simulink model "DRPLDM"  (R2019a)
settings: Solver=FixedStepAuto  StartTime=0.0  StopTime=TimeVector(end)  FixedStep=Tsim  RelTol=1e-3  EnableMultiTasking=on
values from neighbouring files (symbols this model uses):
  Ad = 0.9048    [RunModel.m]
  B1DELTT = [1 100 130]    [RunModel.m]
  B1ERPM = [0 20000 23000]    [RunModel.m]
  B1NOOILT = [300 450 573]    [RunModel.m]
  B2DELTT = [1 40 120]    [RunModel.m]
  B2ERPM = [0 20000 23000]    [RunModel.m]
  B2NOOILT = [300 400 530]    [RunModel.m]
  B3DELTT = [1 50 110]    [RunModel.m]
  B3ERPM = [0 20000 23000]    [RunModel.m]
  B3NOOILT = [300 410 540]    [RunModel.m]
  Bd = 0.1903    [RunModel.m]
  BoosterVec = [hex2dec('55'), hex2dec('AA') hex2dec('FF')]    [RunModel.m]
  Cd = -0.5    [RunModel.m]
  Dd = 0    [RunModel.m]
  DigKeys = bin2dec('0101011')    [RunModel.m]
  EngUnits = 1    [RunModel.m]
  ExComTime = ExComTime + DeltaTimeEnd    [RunModel.m]
  ExComVec = [hex2dec('AA'), hex2dec('00'), hex2dec('CC')]    [RunModel.m]
  ExtFPModel = 0    [RunModel.m]
  FlightStart = 0    [RunModel.m]
  HILMode = 1    [RunModel.m]
  LeverMode = 1    [RunModel.m]
  Mode = 0    [RunModel.m]
  Mwm = 0.35    [RunModel.m]
  OPRPMMax = 4500    [RunModel.m]
  SensFaultStartTime = SensFaultStartTime + DeltaTimeEnd    [RunModel.m]
  SensFaultStopTime = SensFaultStopTime + DeltaTimeEnd    [RunModel.m]
  SysFaultStartTime = SysFaultStartTime + DeltaTimeEnd    [RunModel.m]
  SysFaultStopTime = SysFaultStopTime + DeltaTimeEnd    [RunModel.m]
  TBear1Init = 0    [RunModel.m]
  TBear2Init = 0    [RunModel.m]
  TBear3Init = 0    [RunModel.m]
  Tsim = 0.001 * TICK    [RunModel.m]
  WhichCont = 2    [RunModel.m]
  WhichEngine = 1    [RunModel.m]
undefined symbols (not defined in the file or in its folder): BiasSens, BoosterLStatusTime, BoosterRStatusTime
libraries: Lib_Solve_ModelSource_TMATS x5, simulink x5
(part 1 of 2)
settings Model: Creator=antoniohadadeneto  LastModifiedBy=anton
settings DataIOCC: ReturnWorkspaceOutputs=off
settings OptimizationCC: LifeSpan=inf
settings DebuggingCC: AllowSymbolicDim=off  SFUnexpectedBacktrackingDiag=warning  SFNoUnconditionalDefaultTransitionDiag=warning  SFExecutionAtInitializationDiag=none  ArithmeticOperatorsInVariantConditions=warning
settings ModelReferenceCC: PropagateSignalLabelsOutOfModel=off
settings SFSimCC: SimUseLocalCustomCode=off
settings RTWCC: RTWUseLocalCustomCode=off
settings CodeAppCC: StateflowObjectComments=on
settings GRTTargetCC: TargetLangStandard=C89/C90 (ANSI)
settings ConfigComp: CovMetricSettings=dw  CovHtmlReporting=on  CovSaveCumulativeToWorkspaceVar=on  CovSaveSingleToWorkspaceVar=on  CovExternalEMLEnable=off

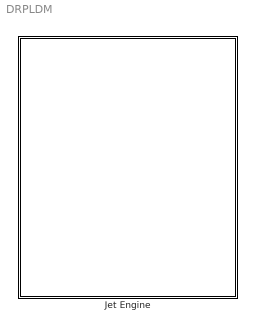
== system DRPLDM ==
  Jet Engine : Subsystem

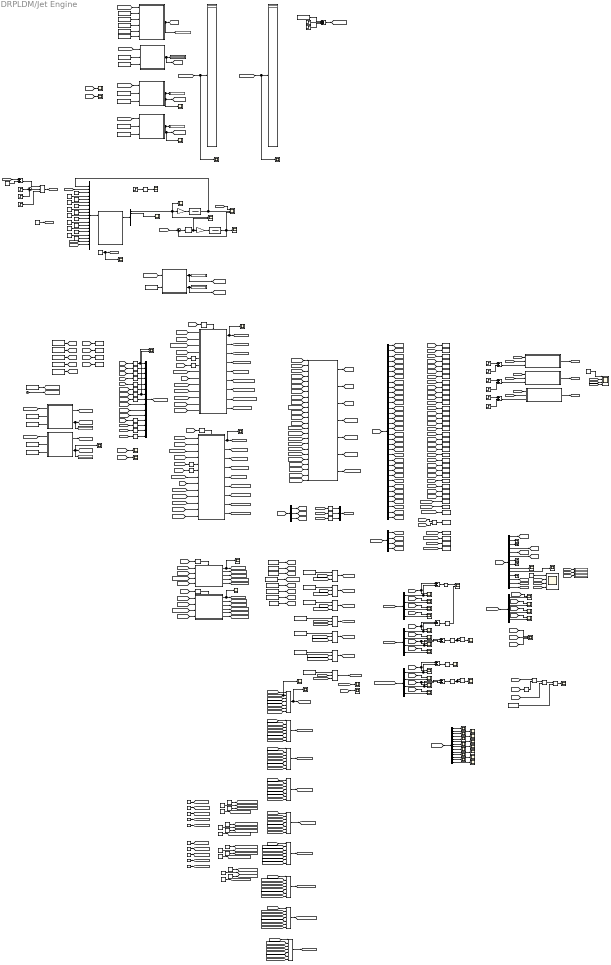
== system DRPLDM/Jet Engine ==
  note: SysFaultTime positions for Emergency and Shut Off respectively
  note: Vector Inputs
  note: Single Spoo Engine
      | Piecewise
      | Linear Model
  note: Bearings Models
  note: Output Selectors
  note: FADEC
  note: To Workspace
  Abnormal DeltaT Bear1 1 : Step  Time=30  After=-50  SampleTime=0
  Abnormal DeltaT Bear1 2 : Step  Time=50  After=50  SampleTime=0
  Abnormal DeltaT Bear2 1 : Step  Time=60  After=0  SampleTime=0
  Abnormal DeltaT Bear2 2 : Step  Time=90  After=0  SampleTime=0
  Abnormal DeltaT Bear3 1 : Step  Time=60  After=0  SampleTime=0
  Abnormal DeltaT Bear3 2 : Step  Time=60  After=0  SampleTime=0
  Abs{,1..4} (5 alike) : Abs
  Add{,1..2,4..5} (5 alike) : Sum  Inputs=+-
  Add{3,9..11} (4 alike) : Sum
  Add6 : Sum  Inputs=+-+
  AltVecDyn : Lib_Solve_ModelSource_TMATS/Model Source  T_vec_M=TimeVector  input_array_M=AltVecDyn
  Bearing 1 : Subsystem
  Bearing 2 : Subsystem
  Bearing 3 : Subsystem
  Bus Creator : BusCreator  Inputs=3
  Bus Creator1 : BusCreator  Inputs=19
  Bus Creator3 : BusCreator  Inputs=15
  Clock : Clock
  Constant{,24,26..32,34,36..41,61..63,65..67,69..78} (32 alike) : Constant
  Constant1 : Constant  Value=Mode
  Constant10 : Constant  Value=SysFaultStartTime
  Constant11 : Constant  Value=BiasSens
  Constant12 : Constant  Value=SensFaultStopTime
  Constant13 : Constant  Value=ExComTime
  Constant14 : Constant  Value=SensFaultStartTime
  Constant15 : Constant  Value=SysFaultStopTime
  Constant16 : Constant  Value=3.1425e-2
  Constant17 : Constant  Value=SysFaultStartTime
  Constant18 : Constant  Value=ExComVec
  Constant19 : Constant  Value=[6 5]
  Constant2 : Constant  Value=LeverMode
  Constant20 : Constant  Value=[30 31]
  Constant{4..5,21..23,42..43} (7 alike) : Constant  Value=HILMode + 1
  Constant25 : Constant  Value=WhichEngine
  Constant3 : Constant  Value=HILMode
  Constant{33,51,53,55..60,64,68} (11 alike) : Constant  Value=0
  Constant35 : Constant  Value=433
  Constant44 : Constant  Value=400
  Constant45 : Constant  Value=3900
  Constant46 : Constant  Value=BoosterLStatusTime
  Constant47 : Constant  Value=BoosterVec
  Constant48 : Constant  Value=BoosterRStatusTime
  Constant49 : Constant  Value=BoosterVec
  Constant50 : Constant  Value=[28 29]
  Constant52 : Constant  Value=ExtFPModel
  Constant54 : Constant  Value=FlightStart
  Constant6 : Constant  Value=EngUnits
  Constant7 : Constant  Value=Mwm
  Constant8 : Constant  Value=DigKeys
  Constant9 : Constant  Value=SysFaultStopTime
  Demux : Demux  Outputs=6
  Demux{1..4,8} (5 alike) : Demux
  Demux5 : Demux  Outputs=3
  Demux6 : Demux  Outputs=34
  Demux7 : Demux  Outputs=14
  Demux9 : Demux  Outputs=14
  Discrete Transfer Fcn : DiscreteTransferFcn  Numerator=0.4866  Denominator=[1 -0.5134]  SampleTime=Tsim
  Discrete Transfer Fcn1 : DiscreteTransferFcn  Numerator=0.4866  Denominator=[1 -0.5134]  SampleTime=Tsim
  Display{,1..12} (13 alike) : Display
  Divide : Product  Inputs=*/
  Divide1 : Product  Inputs=*/
  Divide2 : Product  Inputs=*/
  GEJ85 FADEC : Subsystem  TreatAsAtomicUnit=on
  Gain : Gain  Gain=3000/5
  Gain1 : Gain  Gain=3000/5
  Interval Test : simulink/Logic and Bit Operations/Interval Test  IntervalClosedRight=on  uplimit=1.5  IntervalClosedLeft=on  lowlimit=0.5  OutDataTypeStr=boolean
  Interval Test1 : simulink/Logic and Bit Operations/Interval Test  IntervalClosedRight=on  uplimit=5.5  IntervalClosedLeft=on  lowlimit=4.5  OutDataTypeStr=boolean
  Interval Test3 : simulink/Logic and Bit Operations/Interval Test  IntervalClosedRight=on  uplimit=2.5  IntervalClosedLeft=on  lowlimit=1.5  OutDataTypeStr=boolean
  Interval Test4 : simulink/Logic and Bit Operations/Interval Test  IntervalClosedRight=on  uplimit=3.5  IntervalClosedLeft=on  lowlimit=2.5  OutDataTypeStr=boolean
  MATLAB Function1 : MATLAB Function  TreatAsAtomicUnit=on
  MATLAB Function2 : MATLAB Function  TreatAsAtomicUnit=on
  MATLAB Function3 : MATLAB Function  TreatAsAtomicUnit=on
  MATLAB Function4 : MATLAB Function  TreatAsAtomicUnit=on
  MATLAB Function5 : MATLAB Function  TreatAsAtomicUnit=on
  MATLAB Function6 : MATLAB Function  TreatAsAtomicUnit=on
  MATLAB Function7 : MATLAB Function  TreatAsAtomicUnit=on
  MNVecDyn : Lib_Solve_ModelSource_TMATS/Model Source  T_vec_M=TimeVector  input_array_M=MNVecDyn
  Memory{1..12,15,17..19,21,24..25} (19 alike) : Memory
  Multiport Switch{,1..4,13..16} (9 alike) : MultiPortSwitch  Inputs=6
  Multiport Switch{5..12} (8 alike) : MultiPortSwitch  Inputs=2
  PID Controller2 : simulink/Continuous/PID Controller  Controller=PI  Form=Parallel  TimeDomain=Discrete-time  SampleTime=Tsim  IntegratorMethod=Forward Euler  FilterMethod=Forward Euler  ControllerParametersSource=internal  P=0.0021179  I=3.6301e-03  D=0  UseFilter=on  N=100  TunerSelectOption=Transfer Function Based (PID Tuner App)  InitialConditionSource=internal  InitialConditionForIntegrator=0  InitialConditionForFilter=0  DifferentiatorICPrevScaledInput=0  ExternalReset=none  TrackingMode=off  Kt=1  LimitOutput=off  UpperSaturationLimit=inf  LowerSaturationLimit=-inf  LinearizeAsGain=on  AntiWindupMode=none  Kb=1  POutMin=[]  POutMax=[]  IOutMin=[]  IOutMax=[]  DOutMin=[]  DOutMax=[]  NOutMin=[]  NOutMax=[]  SumOutMin=[]  SumOutMax=[]  SaturationOutMin=[]  SaturationOutMax=[]  PParamMin=[]  PParamMax=[]  IParamMin=[]  IParamMax=[]  DParamMin=[]  DParamMax=[]  NParamMin=[]  NParamMax=[]  KbParamMin=[]  KbParamMax=[]  KtParamMin=[]  KtParamMax=[]  KbOutMin=[]  KbOutMax=[]  KtOutMin=[]  KtOutMax=[]  IntegratorOutMin=[]  IntegratorOutMax=[]  FilterOutMin=[]  FilterOutMax=[]  SumI1OutMin=[]  SumI1OutMax=[]  SumI2OutMin=[]  SumI2OutMax=[]  SumI3OutMin=[]  SumI3OutMax=[]  SumI4OutMin=[]  SumI4OutMax=[]  SumDOutMin=[]  SumDOutMax=[]  DifferentiatorOutMin=[]  DifferentiatorOutMax=[]  FilterDiffOutCoefMin=[]  FilterDiffOutCoefMax=[]  ReciprocalOutMin=[]  ReciprocalOutMax=[]  SumDenOutMin=[]  SumDenOutMax=[]  SumNumOutMin=[]  SumNumOutMax=[]  DivideOutMin=[]  DivideOutMax=[]  IntegratorContinuousStateAttributes=''  IntegratorStateMustResolveToSignalObject=off  IntegratorRTWStateStorageClass=Auto  FilterContinuousStateAttributes=''  FilterStateMustResolveToSignalObject=off  FilterRTWStateStorageClass=Auto  ParallelPVariant=InternalParameters  IdealPVariant=Disabled  IVariant=InternalParameters  DVariant=Disabled  IntegratorVariant=Discrete  SatVariant=Disabled  AWVariant=Passthrough  PCopyVariant=Disabled  TRVariant=Disabled  FdbkBlocksVariant=Forward  IdealPFdbkVariant=Disabled  SatFdbkVariant=Disabled  DerivativeFilterVariant=Disabled  NVariant=Disabled  NCopyVariant=Disabled_SignalSpec  FilterICVariant=Disabled  IntegratorICVariant=InternalICs  ExternalResetVariant=Disabled  TRSumVariant=Passthrough  SumFdbkVariant=Disabled  SumVariant=Sum_PI
  Product : Product
  Product1 : Product
  Product2 : Product
  Pulse Generator1 : DiscretePulseGenerator  PulseType=Time based  Period=2 * 0.001 * 200  PulseWidth=50
  Rate Limiter1 : RateLimiter  RisingSlewLimit=2  FallingSlewLimit=-2  SampleTimeMode=inherited
  RefVecDyn : Lib_Solve_ModelSource_TMATS/Model Source  T_vec_M=TimeVector  input_array_M=RefVecDyn
  Reset Input : Lib_Solve_ModelSource_TMATS/Model Source  T_vec_M=TimeVector  input_array_M=ResetInput
  S-Function2 : S-Function  FunctionName=FuelPumpCL_TJ1200_TestBench  SFunctionDeploymentMode=off  EnableBusSupport=off
  Scope{,1..6,10,17..20,27..30,32,34..35,40,42..55,57..64} (42 alike) : Scope
  Scope{7..9,11..16,21..24,31,36..39,56} (19 alike) : Scope  NumInputPorts=2
  Scope25 : Scope  NumInputPorts=3
  Scope26 : Scope  NumInputPorts=3
  Scope33 : Scope  NumInputPorts=4
  Scope41 : Scope  NumInputPorts=4
  Single Spool Engine : Subsystem  TreatAsAtomicUnit=on
  Sqrt : Sqrt  SaturateOnIntegerOverflow=on
  Step : Step  Time=40  After=1000  SampleTime=0
  Step1 : Step  Time=60  After=1000  SampleTime=0
  Step2 : Step  After=2000  SampleTime=0
  Step3 : Step  After=2750  SampleTime=0
  Step4 : Step  Time=10  After=-1000  SampleTime=0
  Step5 : Step  After=5  SampleTime=0
  Sum : Sum  Inputs=|++
  Sum1 : Sum  Inputs=|+-
  TF1200 FADEC : Subsystem  TreatAsAtomicUnit=on
  TJ1200 FADEC : Subsystem  TreatAsAtomicUnit=on
  TJ1200 FADEC1 : Subsystem  TreatAsAtomicUnit=on
  Terminator{,3..4,8..9} (5 alike) : Terminator
  To Workspace1 : ToWorkspace  VariableName=Active_HIL  SampleTime=-1
  To Workspace10 : ToWorkspace  VariableName=MN  SampleTime=-1
  To Workspace11 : ToWorkspace  VariableName=Ref  SampleTime=-1
  To Workspace12 : ToWorkspace  VariableName=RU_HIL  SampleTime=-1
  To Workspace13 : ToWorkspace  VariableName=N_HIL  SampleTime=-1
  To Workspace14 : ToWorkspace  VariableName=Pt5_HIL  SampleTime=-1
  To Workspace15 : ToWorkspace  VariableName=Tt5_HIL  SampleTime=-1
  To Workspace17 : ToWorkspace  VariableName=Tt4_HIL  SampleTime=-1
  To Workspace18 : ToWorkspace  VariableName=Pt3_HIL  SampleTime=-1
  To Workspace2 : ToWorkspace  VariableName=RPMRef_HIL  SampleTime=-1
  To Workspace21 : ToWorkspace  VariableName=PRFAN_HIL  SampleTime=-1
  To Workspace22 : ToWorkspace  VariableName=WcFAN_HIL  SampleTime=-1
  To Workspace23 : ToWorkspace  VariableName=Pt21_HIL  SampleTime=-1
  To Workspace24 : ToWorkspace  VariableName=Fn_HIL  SampleTime=-1
  To Workspace25 : ToWorkspace  VariableName=Wf_HIL  SampleTime=-1
  To Workspace26 : ToWorkspace  VariableName=Fg_HIL  SampleTime=-1
  To Workspace27 : ToWorkspace  VariableName=POil_HIL  SampleTime=-1
  To Workspace28 : ToWorkspace  VariableName=Ignition_HIL  SampleTime=-1
  To Workspace29 : ToWorkspace  VariableName=V8_HIL  SampleTime=-1
  To Workspace3 : ToWorkspace  VariableName=FiltRef_HIL  SampleTime=-1
  To Workspace30 : ToWorkspace  VariableName=W8_HIL  SampleTime=-1
  To Workspace31 : ToWorkspace  VariableName=Tt6_HIL  SampleTime=-1
  To Workspace32 : ToWorkspace  VariableName=Pt6_HIL  SampleTime=-1
  To Workspace33 : ToWorkspace  VariableName=Tt3_HIL  SampleTime=-1
  To Workspace34 : ToWorkspace  VariableName=SMHPC_HIL  SampleTime=-1
  To Workspace35 : ToWorkspace  VariableName=WcHPC_HIL  SampleTime=-1
  To Workspace36 : ToWorkspace  VariableName=PRHPC_HIL  SampleTime=-1
  To Workspace37 : ToWorkspace  VariableName=NcHPC_HIL  SampleTime=-1
  To Workspace38 : ToWorkspace  VariableName=Tt21_HIL  SampleTime=-1
  To Workspace39 : ToWorkspace  VariableName=SMFAN_HIL  SampleTime=-1
  To Workspace4 : ToWorkspace  VariableName=QSMCdy_HIL  SampleTime=-1
  To Workspace40 : ToWorkspace  VariableName=BPFAN_HIL  SampleTime=-1
  To Workspace41 : ToWorkspace  VariableName=W21_HIL  SampleTime=-1
  To Workspace42 : ToWorkspace  VariableName=NcFAN_HIL  SampleTime=-1
  To Workspace43 : ToWorkspace  VariableName=Pt2_HIL  SampleTime=-1
  To Workspace44 : ToWorkspace  VariableName=Tt2_HIL  SampleTime=-1
  To Workspace45 : ToWorkspace  VariableName=W2_HIL  SampleTime=-1
  To Workspace5 : ToWorkspace  VariableName=QSMCdx_HIL  SampleTime=-1
  To Workspace6 : ToWorkspace  VariableName=QSMCuy_HIL  SampleTime=-1
  To Workspace7 : ToWorkspace  VariableName=QSMCux_HIL  SampleTime=-1
  To Workspace8 : ToWorkspace  VariableName=dT  SampleTime=-1
  To Workspace9 : ToWorkspace  VariableName=Altitude  SampleTime=-1
  dTVecDyn : Lib_Solve_ModelSource_TMATS/Model Source  T_vec_M=TimeVector  input_array_M=dTVecDyn
  wires:
  [QSMC_uy] -> To Workspace6/1
  Demux6/29 -> [POil_HIL]
  [Pt5_HIL] -> To Workspace14/1
  Demux6/16 -> [Pt3_HIL]
  [Fn_HIL] -> To Workspace24/1
  [Reset_HIL] -> Single Spool Engine/7(Reset)
  Demux6/15 -> [SMHPC_HIL]
  [WhichEngine] -> Interval Test3/1
  [Wf_HIL] -> To Workspace25/1
  dTVecDyn/1 -> [dT]
  GEJ85 FADEC/2(Active Controller) -> [Active_GEJ85FADEC]
  [Pt3_HIL] -> To Workspace18/1
  Memory19/1 -> Scope56/1, Bus Creator3/1  "N"
  [WcFAN_HIL] -> To Workspace22/1
  [NcHPC_HIL] -> To Workspace37/1
  [Tt3_HIL] -> To Workspace33/1
  [Active_HIL] -> To Workspace1/1
  Interval Test3/1 -> TF1200 FADEC/Enable
  [W21_HIL] -> To Workspace41/1
  [WhichEngine] -> Interval Test/1
  Demux6/30 -> [Ignition_HIL]
  Interval Test/1 -> TJ1200 FADEC/Enable
  [Ignition_HIL] -> To Workspace28/1
  [Pt2_HIL] -> To Workspace43/1
  Constant2/1 -> [LeverMode]
  Memory1/1 -> Bus Creator3/12  "Pt2"
  [MN] -> TJ1200 FADEC/2(MN)
  [QSMC_dxy] -> Demux1/1
  TJ1200 FADEC/3(Igniter) -> [Igniter_TJ1200FADEC]
  [Tt21_HIL] -> To Workspace38/1
  GEJ85 FADEC/4(RPMRef) -> [RPMRef_GEJ85FADEC]
  Demux6/31 -> [RPMRef_SIL]
  Multiport Switch2/1 -> [Igniter_FADEC]
  Demux6/22 -> [Pt6_HIL]
  Constant3/1 -> [HILMode]
  Demux6/21 -> [Tt5_HIL]
  Demux6/17 -> [Tt3_HIL]
  [Pt6_HIL] -> To Workspace32/1
  Demux6/25 -> [V8_HIL]
  [Ref] -> Single Spool Engine/6(SoftLoop Ref)
  [Output] -> Demux6/1
  [N_HIL] -> To Workspace13/1
  Demux6/3 -> [Tt2_HIL]
  Demux6/32 -> [FiltRef_SIL]
  Demux6/23 -> [Tt6_HIL]
  Demux6/13 -> [WcHPC_HIL]
  Memory12/1 -> Bus Creator3/8  "Wf0"
  Multiport Switch/1 -> Scope62/1, [Wf_FADEC]
  Memory21/1 -> Bus Creator3/2  "Pt3"
  TJ1200 FADEC/2(Active Controller) -> [Active_TJ1200FADEC]
  Demux6/24 -> [W8_HIL]
  Demux6/19 -> [Wf_HIL]
  [WhichEngine] -> Multiport Switch2/1
  [SMHPC_HIL] -> To Workspace34/1
  [Igniter_TJ1200FADEC] -> Multiport Switch2/2
  Demux6/26 -> [Fn_HIL]
  [Altitude] -> GEJ85 FADEC/1(Altitude)
  [ControlIn] -> TJ1200 FADEC/3(Engine Outputs)
  [Tt6_HIL] -> To Workspace31/1
  [PRHPC_HIL] -> To Workspace36/1
  [NcFAN_HIL] -> To Workspace42/1
  [W2_HIL] -> To Workspace45/1
  [ControlIn] -> TF1200 FADEC/3(Engine Outputs)
  [Tt2_HIL] -> To Workspace44/1
  Interval Test4/1 -> GEJ85 FADEC/Enable
  [FiltRef_TJ1200FADEC] -> Multiport Switch4/2
  [RPMRef_TF1200FADEC] -> Multiport Switch3/3
  Demux5/1 -> [Wf0_HIL]
  [Pt3_HIL] -> Memory21/1
  [Ref] -> TJ1200 FADEC/4(RefVecDyn)
  [ControlIn] -> GEJ85 FADEC/3(Engine Outputs)
  TJ1200 FADEC/1(MinMaxWf) -> Scope2/1, [Wf_TJ1200FADEC]
  [Altitude] -> TJ1200 FADEC/1(Altitude)
  Constant25/1 -> [WhichEngine]
  [LeverMode] -> Bus Creator3/11  "LeverMode"
  Memory25/1 -> Scope56/2, Bus Creator3/7  "Authorize"
  [Mode] -> Bus Creator3/10  "Mode"
  [Reset_HIL] -> Bus Creator3/9  "Reset"
  [W8_HIL] -> To Workspace30/1
  [V8_HIL] -> To Workspace29/1
  TF1200 FADEC/1(MinMaxWf) -> Scope/1, [Wf_TF1200FADEC]
  [SMFAN_HIL] -> To Workspace39/1
  Memory15/1 -> Bus Creator3/5  "POil"
  Demux6/28 -> [N_HIL]
  [Wf0_HIL] -> Memory12/1
  TF1200 FADEC/2(Active Controller) -> [Active_TF1200FADEC]
  Demux5/2 -> [SkSt_HIL]
  Demux6/6 -> [PRFAN_HIL]
  [Ref] -> TF1200 FADEC/4(RefVecDyn)
  Memory17/1 -> Bus Creator3/4  "Tt2"
  TF1200 FADEC/3(Igniter) -> [Igniter_TF1200FADEC]
  [N_HIL] -> Memory19/1
  [MN] -> GEJ85 FADEC/2(MN)
  [MN] -> TF1200 FADEC/2(MN)
  Demux6/10 -> [Pt21_HIL]
  GEJ85 FADEC/3(Igniter) -> [Igniter_GEJ85FADEC]
  Demux6/11 -> [Tt21_HIL]
  MNVecDyn/1 -> [MN]
  AltVecDyn/1 -> [Altitude]
  Demux6/12 -> [NcHPC_HIL]
  [RPMRef_TJ1200FADEC] -> Multiport Switch3/2
  [Altitude] -> TF1200 FADEC/1(Altitude)
  Single Spool Engine/1(Outputs) -> [Output]
  [dT] -> Single Spool Engine/3(dT)
  Constant5/1 -> Multiport Switch6/1
  [Tt5_HIL] -> To Workspace15/1
  [Pt21_HIL] -> To Workspace23/1
  [Tt4_HIL] -> To Workspace17/1
  [PRFAN_HIL] -> To Workspace21/1
  [Wf_FADEC] -> Single Spool Engine/4(Wf)
  [Altitude] -> Single Spool Engine/1(Altitude)
  Demux6/1 -> [W2_HIL]
  Demux6/5 -> [WcFAN_HIL]
  [Fg_HIL] -> To Workspace26/1
  Demux6/9 -> [W21_HIL]
  [Mode] -> Single Spool Engine/8(Mode)
  Demux1/3 -> [QSMC_ux]
  [FiltRef_GEJ85FADEC] -> Multiport Switch4/4
  [WhichEngine] -> Interval Test4/1
  [Wf_TF1200FADEC] -> Multiport Switch/3
  TF1200 FADEC/5(FiltRef) -> [FiltRef_TF1200FADEC]
  Constant4/1 -> Multiport Switch5/1
  [WhichEngine] -> Multiport Switch4/1
  [Wf_TJ1200FADEC] -> Scope63/1, Multiport Switch/2
  Reset Input/1 -> [Reset_HIL]
  [WhichEngine] -> Multiport Switch3/1
  [WhichEngine] -> Multiport Switch1/1
  [Active_TF1200FADEC] -> Multiport Switch1/3
  [Active_GEJ85FADEC] -> Multiport Switch1/4
  [WhichEngine] -> Multiport Switch/1
  [SkSt_HIL] -> Memory18/1
  [MN] -> Single Spool Engine/2(MN)
  [FiltRef_SIL] -> Multiport Switch6/2
  Memory24/1 -> Bus Creator3/3  "Tt5"
  [RPMRef_SIL] -> Multiport Switch5/2
  Demux5/3 -> [Atrz_HIL]
  [Igniter_FADEC] -> Single Spool Engine/5(Ignition)
  [FiltRef_HIL] -> To Workspace3/1
  [RPMRef_FADEC] -> Multiport Switch5/3
  [WhichEngine] -> Single Spool Engine/11(WhichEngine)
  [Active_TJ1200FADEC] -> Multiport Switch1/2
  [FiltRef_TF1200FADEC] -> Multiport Switch4/3
  [FiltRef_FADEC] -> Multiport Switch6/3
  GEJ85 FADEC/5(FiltRef) -> [FiltRef_GEJ85FADEC]
  TJ1200 FADEC/4(RPMRef) -> [RPMRef_TJ1200FADEC]
  [Igniter_TF1200FADEC] -> Multiport Switch2/3
  TF1200 FADEC/4(RPMRef) -> [RPMRef_TF1200FADEC]
  [POil_HIL] -> To Workspace27/1
  Demux6/7 -> [SMFAN_HIL]
  Demux6/20 -> [Pt5_HIL]
  [WcHPC_HIL] -> To Workspace35/1
  [Ref] -> GEJ85 FADEC/4(RefVecDyn)
  GEJ85 FADEC/1(MinMaxWf) -> Scope1/1, [Wf_GEJ85FADEC]
  Multiport Switch6/1 -> [FiltRef_HIL]
  Multiport Switch3/1 -> [RPMRef_FADEC]
  [Tt5_HIL] -> Memory24/1
  Multiport Switch5/1 -> [RPMRef_HIL]
  [Wf_GEJ85FADEC] -> Multiport Switch/4
  [BPFAN_HIL] -> To Workspace40/1
  Demux6/8 -> [BPFAN_HIL]
  [Atrz_HIL] -> Memory25/1
  Demux6/27 -> [Fg_HIL]
  [Igniter_GEJ85FADEC] -> Multiport Switch2/4
  [RPMRef_GEJ85FADEC] -> Multiport Switch3/4
  [Tt2_HIL] -> Memory17/1
  [QSMC_dy] -> To Workspace4/1
  RefVecDyn/1 -> [Ref]
  Demux1/2 -> [QSMC_dy]
  Demux6/18 -> [Tt4_HIL]
  Demux6/4 -> [NcFAN_HIL]
  Multiport Switch1/1 -> [Active_FADEC]
  Constant1/1 -> [Mode]
  [QSMC_dx] -> To Workspace5/1
  Single Spool Engine/2(InitOut) -> [InitOut]
  Demux6/2 -> [Pt2_HIL]
  [QSMC_ux] -> To Workspace7/1
  GEJ85 FADEC/6(QSMC_dxy) -> [QSMC_dxy]
  Demux1/1 -> [QSMC_dx]
  [InitOut] -> Demux5/1
  Demux1/4 -> [QSMC_uy]
  TJ1200 FADEC/5(FiltRef) -> [FiltRef_TJ1200FADEC]
  Bus Creator3/1 -> [ControlIn]
  Multiport Switch4/1 -> [FiltRef_FADEC]
  [LeverMode] -> Single Spool Engine/9(LeverMode)
  [Pt2_HIL] -> Memory1/1
  Memory18/1 -> Bus Creator3/6  "SkipStart"
  [POil_HIL] -> Memory15/1
  [RPMRef_HIL] -> To Workspace2/1
  Demux6/14 -> [PRHPC_HIL]
  [HILMode] -> Single Spool Engine/10(HILMode)
  Constant6/1 -> [EngUnits]
  [EngUnits] -> Single Spool Engine/12(EngUhits)
  [Mwm] -> Single Spool Engine/13(Windmill Mach Number)
  Constant7/1 -> [Mwm]
  Single Spool Engine/3(Sensors) -> [Sensors]
  [Sensors] -> Memory2/1
  Memory2/1 -> TJ1200 FADEC/5(Sensors)
  Memory3/1 -> TJ1200 FADEC/6(Tt4)  "Tt4"
  [Tt4_HIL] -> Memory3/1
  Clock/1 -> [Time]
  [SensFaults] -> TJ1200 FADEC/7(Sensor Faults)
  Constant11/1 -> [Bias]
  [Bias] -> Single Spool Engine/14(Bias)
  Constant14/1 -> MATLAB Function2/2(StartTime)
  Constant12/1 -> MATLAB Function2/3(StopTime)
  [Time] -> MATLAB Function2/1(Time)
  MATLAB Function2/2(IntRep) -> Display1/1, [SensFaults]
  MATLAB Function2/1(Bits) -> [SensFaultBits]
  [SensFaultBits] -> Display3/1, Scope4/1
  MATLAB Function3/1(Bits) -> [SysFaultBits]
  MATLAB Function3/2(IntRep) -> Scope6/1, Display4/1, [SysFaults]
  Constant15/1 -> MATLAB Function3/3(StopTime)
  Constant17/1 -> MATLAB Function3/2(StartTime)
  [Time] -> MATLAB Function3/1(Time)
  [SensFaults] -> Single Spool Engine/15(Sensor Faults)
  [SysFaults] -> Single Spool Engine/16(System Faults)
  [SysFaultBits] -> Scope3/1, Display2/1
  MATLAB Function1/1(DigKeysOut) -> Display5/1, [DigKeys]
  [DigKeys] -> TJ1200 FADEC/8(Digital Keys)
  [Time] -> MATLAB Function1/1(Time)
  Constant10/1 -> MATLAB Function1/2(StartTime)
  Constant9/1 -> MATLAB Function1/3(StopTime)
  Constant8/1 -> MATLAB Function1/4(DigKeysIn)
  [Time] -> MATLAB Function4/1(Time)
  Constant13/1 -> MATLAB Function4/2(ExComTime)
  MATLAB Function4/1(Output) -> [ExCom], Display6/1
  [Reset_HIL] -> Scope5/1
  Constant19/1 -> MATLAB Function1/5(BitPosition)
  Constant20/1 -> MATLAB Function1/6(TimePosition)
  TJ1200 FADEC/6(Normal Model) -> [NormalModel_TJ1200FADEC]
  TJ1200 FADEC/7(Fuel Lack Model) -> [FuelLackModel_TJ1200FADEC]
  Abs/1 -> Scope16/1
  [Wf_HIL] -> Scope11/1  "Nmech"
  Product/1 -> Scope10/1
  Add1/1 -> Abs1/1
  Add2/1 -> Abs2/1
  Add/1 -> Abs/1
  Abs1/1 -> Scope16/2
  Demux3/4 -> Scope11/2
  [N_HIL] -> Add1/1, Scope12/1  "Nmech"
  Demux3/3 -> Scope9/2
  [NormalModel] -> Demux3/1
  Demux4/1 -> Add1/2, Scope12/2
  Demux4/3 -> Add2/2, Scope14/2
  Demux4/2 -> Scope13/2
  [FuelLackModel] -> Demux4/1
  [Pt3_HIL] -> Add2/1, Scope14/1  "Nmech"
  [Tt4_HIL] -> Scope13/1  "Nmech"
  [Pt3_HIL] -> Scope9/1  "Nmech"
  Abs2/1 -> Product/1, Product/2
  Demux3/1 -> Add/2, Scope7/2
  [Tt2_HIL] -> Scope15/1  "Nmech"
  Demux3/2 -> Scope8/2
  [Tt4_HIL] -> Scope8/1  "Nmech"
  [N_HIL] -> Add/1, Scope7/1  "Nmech"
  [Tt5_HIL] -> Sqrt/1  "Nmech"
  [W8_HIL] -> Product1/1  "Nmech"
  Sqrt/1 -> Product1/2
  Product1/1 -> Divide/1
  [Pt5_HIL] -> Divide/2  "Nmech"
  Divide/1 -> Divide1/1
  Constant16/1 -> Divide1/2
  Divide1/1 -> Scope17/1
  [Wf0_HIL] -> Scope18/1
  Constant18/1 -> MATLAB Function4/3(Command)
  [ExCom] -> Single Spool Engine/17(ExCom (Start/ShutDown))
  Demux6/33 -> [Active_SIL]
  Multiport Switch7/1 -> [Active_HIL]
  [Active_FADEC] -> Multiport Switch7/3
  [Active_SIL] -> Multiport Switch7/2
  Constant21/1 -> Multiport Switch7/1
  [ExCom] -> TJ1200 FADEC/9(OnOffCom)
  [SkSt_HIL] -> Scope19/1
  [SkSt_HIL] -> Scope20/1
  Constant22/1 -> Multiport Switch8/1
  [NormalModel_SIL] -> Multiport Switch8/2
  [NormalModel_FADEC] -> Multiport Switch8/3
  Multiport Switch8/1 -> [NormalModel]
  Multiport Switch9/1 -> [FuelLackModel]
  [FuelLackModel_FADEC] -> Multiport Switch9/3
  [FuelLackModel_SIL] -> Multiport Switch9/2
  Constant23/1 -> Multiport Switch9/1
  Single Spool Engine/4(NormalModel) -> [NormalModel_SIL]
  Single Spool Engine/5(FuelLackModel) -> [FuelLackModel_SIL]
  Single Spool Engine/6(SensorModel) -> [SensorModel]
  [SensorModel] -> Demux2/1
  Demux2/1 -> Scope21/2
  Demux2/2 -> Scope22/2
  Demux2/3 -> Scope23/2
  [Tt4_HIL] -> Scope23/1  "Nmech"
  [Pt3_HIL] -> Scope22/1  "Nmech"
  [Sensors] -> Demux7/1
  Demux7/11 -> Terminator/1
  Demux7/10 -> Scope60/1
  Demux7/8 -> Terminator3/1
  Demux7/9 -> Scope59/1
  Demux7/4 -> [Tt4Sensor0]
  Demux7/5 -> [Tt4Sensor1]
  Demux7/6 -> [Tt4Sensor2]
  Demux7/7 -> Terminator4/1
  Demux7/1 -> [Ts2Sensor]
  Demux7/2 -> Terminator9/1
  Demux7/3 -> Terminator8/1
  [Ts2Sensor] -> Scope21/1
  [Wf_HIL] -> Scope24/1  "Nmech"
  Demux2/4 -> Scope24/2
  [Tt4Sensor1] -> Scope25/2
  [Tt4Sensor2] -> Scope25/3
  [Tt4Sensor0] -> Scope25/1
  Gain/1 -> Discrete Transfer Fcn/1
  Discrete Transfer Fcn/1 -> Bus Creator1/1, Scope26/2
  Discrete Transfer Fcn1/1 -> Scope26/3, Scope27/1, Sum1/2
  Gain1/1 -> Discrete Transfer Fcn1/1
  Demux/1 -> Scope30/1, Scope31/1, Gain/1
  Rate Limiter1/1 -> Scope28/1
  Step2/1 -> Rate Limiter1/1
  Bus Creator1/1 -> S-Function2/1
  Constant37/1 -> Bus Creator1/4
  Step3/1 -> Sum/1
  Constant36/1 -> Bus Creator1/3
  Constant39/1 -> Bus Creator1/6
  Constant41/1 -> Bus Creator1/8
  Constant38/1 -> Bus Creator1/5
  Constant40/1 -> Bus Creator1/7
  Constant/1 -> Bus Creator1/9
  Constant24/1 -> Bus Creator1/10
  Constant26/1 -> Bus Creator1/11
  Constant27/1 -> Bus Creator1/12
  Constant28/1 -> Bus Creator1/13
  Constant29/1 -> Bus Creator1/14
  Constant30/1 -> Bus Creator1/15
  Constant31/1 -> Bus Creator1/16
  Constant32/1 -> Bus Creator1/17
  Constant33/1 -> [ModeFP]
  [TickTack] -> Bus Creator1/19
  Pulse Generator1/1 -> Scope29/1, [TickTack]
  S-Function2/1 -> Demux/1
  Sum1/1 -> PID Controller2/1
  [RefFP] -> Sum1/1
  PID Controller2/1 -> Scope31/2, Gain1/1
  Step4/1 -> Sum/2
  Sum/1 -> Multiport Switch10/2
  Step5/1 -> Multiport Switch10/3
  [ModeFP] -> Bus Creator1/18
  [ModeFP] -> Add3/1
  Constant34/1 -> Add3/2
  Add3/1 -> Multiport Switch10/1
  Multiport Switch10/1 -> [RefFP]
  [RefFP] -> Bus Creator1/2
  [RefFP] -> Scope26/1
  Demux/2 -> Scope32/1
  Abnormal DeltaT Bear1 1/1 -> Add9/1
  Bearing 1/1(Bearing Measured Temperature) -> [TBearing1]
  [OPRPM] -> Bearing 1/2(Oil Pump RPM)
  Abnormal DeltaT Bear3 1/1 -> Add11/1
  Abnormal DeltaT Bear3 2/1 -> Add11/2
  [N_HIL] -> Bearing 3/1(Engine RPM)
  Abnormal DeltaT Bear2 2/1 -> Add10/2
  Bearing 3/1(Bearing Measured Temperature) -> [TBearing3]
  Add10/1 -> Bearing 2/3(Abnormal DeltaT)
  Abnormal DeltaT Bear1 2/1 -> Add9/2
  [N_HIL] -> Bearing 2/1(Engine RPM)
  [TBearing3] -> Scope33/4
  Add9/1 -> Bearing 1/3(Abnormal DeltaT)
  [TBearing1] -> Scope33/2
  [OPRPM] -> Bearing 2/2(Oil Pump RPM)
  Constant35/1 -> Scope33/1
  Abnormal DeltaT Bear2 1/1 -> Add10/1
  [OPRPM] -> Bearing 3/2(Oil Pump RPM)
  [N_HIL] -> Bearing 1/1(Engine RPM)
  [TBearing2] -> Scope33/3
  Bearing 2/1(Bearing Measured Temperature) -> [TBearing2]
  Add11/1 -> Bearing 3/3(Abnormal DeltaT)
  [TBearSens0] -> Memory4/1
  [TBearSens2] -> Memory6/1
  [TBearSens1] -> Memory5/1
  Memory4/1 -> Bus Creator3/13  "TBear1"
  Memory5/1 -> Bus Creator3/14  "TBear2"
  Memory6/1 -> Bus Creator3/15  "TBear3"
  TJ1200 FADEC/9(Oil Pump RPM Ref) -> [OPRPM_TJ1200FADEC]
  [TBearing1] -> Memory7/1
  [TBearing3] -> Memory9/1
  [TBearing2] -> Memory8/1
  Bus Creator/1 -> [TBear]
  [TBear] -> Single Spool Engine/18(Bearings Temp)
  Memory7/1 -> Bus Creator/1  "TBear1"
  Memory8/1 -> Bus Creator/2  "TBear2"
  Memory9/1 -> Bus Creator/3  "TBear3"
  Constant42/1 -> Multiport Switch11/1
  [OPRPM_SIL] -> Multiport Switch11/2
  [OPRPM_FADEC] -> Multiport Switch11/3
  Multiport Switch11/1 -> [OPRPM]
  Demux6/34 -> [OPRPM_SIL]
  [OPRPM] -> Scope34/1
  TJ1200 FADEC/8(Closed Loop Model) -> [ClosedLoopModel_TJ1200FADEC]
  [Tt2_HIL] -> Scope39/1  "Nmech"
  Abs4/1 -> Product2/2, Product2/1
  [Tt4_HIL] -> Scope37/1  "Nmech"
  [Fn_HIL] -> Scope38/1, Add5/1  "Nmech"
  [ClosedLoopModel] -> Demux8/1
  Demux8/4 -> Scope39/2
  Demux8/2 -> Scope37/2
  Demux8/3 -> Scope38/2, Add5/2
  Demux8/1 -> Scope36/2, Add4/2
  [N_HIL] -> Scope36/1, Add4/1  "Nmech"
  Add5/1 -> Abs4/1
  Add4/1 -> Abs3/1
  Product2/1 -> Scope35/1
  Abs3/1 -> Scope40/1
  Constant43/1 -> Multiport Switch12/1
  [ClosedLoopModel_SIL] -> Multiport Switch12/2
  [ClosedLoopModel_FADEC] -> Multiport Switch12/3
  Multiport Switch12/1 -> [ClosedLoopModel]
  Single Spool Engine/7(Closed Loop Model) -> [ClosedLoopModel_SIL]
  Demux7/12 -> [TBearSens0]
  Demux7/13 -> [TBearSens1]
  Demux7/14 -> [TBearSens2]
  Constant44/1 -> Scope41/1
  [OPRPM_FADEC] -> Single Spool Engine/19(Oil Pump RPM)
  [TBearSens0] -> Scope41/2
  [TBearSens1] -> Scope41/3
  [TBearSens2] -> Scope41/4
  [Sensors] -> Demux9/1
  Demux9/1 -> Scope44/1
  Demux9/3 -> Scope42/1
  Demux9/7 -> Scope46/1
  Demux9/5 -> Scope47/1
  Demux9/11 -> Scope43/1
  Demux9/9 -> Scope45/1
  Demux9/13 -> Scope48/1
  Demux9/2 -> Scope49/1
  Demux9/4 -> Scope50/1
  Demux9/6 -> Scope51/1
  Demux9/8 -> Scope52/1
  Demux9/10 -> Scope53/1
  Demux9/12 -> Scope54/1
  Demux9/14 -> Scope55/1
  [OPRPMManual] -> Single Spool Engine/20(Oil Pump RPM Manual Ref)
  Constant45/1 -> Add6/1
  [OPRPMManual] -> TJ1200 FADEC/10(Oil Pump RPM Manual Ref)
  Step/1 -> Add6/2
  Step1/1 -> Add6/3
  Add6/1 -> [OPRPMManual]
  [SysFaults] -> TJ1200 FADEC/11(System Faults)
  Constant47/1 -> MATLAB Function5/3(Command)
  MATLAB Function5/1(Output) -> Display7/1, Scope57/1, [BoosterLStatus]
  Constant46/1 -> MATLAB Function5/2(ExComTime)
  [Time] -> MATLAB Function5/1(Time)
  [Time] -> MATLAB Function6/1(Time)
  Constant48/1 -> MATLAB Function6/2(ExComTime)
  MATLAB Function6/1(Output) -> Scope58/1, [BoosterRStatus], Display8/1
  Constant49/1 -> MATLAB Function6/3(Command)
  [BoosterLStatus] -> Single Spool Engine/21(Left Booster Status)
  [BoosterRStatus] -> Single Spool Engine/22(Right Booster Status)
  [BoosterLStatus] -> TJ1200 FADEC/12(Left Booster State)
  [BoosterRStatus] -> TJ1200 FADEC/13(Right Booster State)
  MATLAB Function7/2(CAN1) -> [CAN1Fault], Display9/1
  [SysFaultBits] -> MATLAB Function7/1(SysFaultBits)
  Constant50/1 -> MATLAB Function7/2(Position)
  MATLAB Function7/1(CAN0) -> [CAN0Fault], Display10/1
  [Ref] -> To Workspace11/1
  [Altitude] -> To Workspace9/1
  [MN] -> To Workspace10/1
  [dT] -> To Workspace8/1
  [Wf_HIL] -> Divide2/1
  [Pt3_HIL] -> Divide2/2
  Divide2/1 -> To Workspace12/1
  [POil_HIL] -> Scope61/1
  Constant51/1 -> [Wf_TJ700FADEC]
  [Wf_TJ700FADEC] -> Multiport Switch/5
  [Wf_TJ200FADEC] -> Multiport Switch/6
  Constant53/1 -> [Active_TJ700FADEC]
  [Active_TJ700FADEC] -> Multiport Switch1/5
  [Active_TJ200FADEC] -> Multiport Switch1/6
  Constant55/1 -> [Igniter_TJ700FADEC]
  [Igniter_TJ700FADEC] -> Multiport Switch2/5
  [Igniter_TJ200FADEC] -> Multiport Switch2/6
  [RPMRef_TJ700FADEC] -> Multiport Switch3/5
  [RPMRef_TJ200FADEC] -> Multiport Switch3/6
  Constant57/1 -> [RPMRef_TJ700FADEC]
  Constant59/1 -> [FiltRef_TJ700FADEC]
  [FiltRef_TJ700FADEC] -> Multiport Switch4/5
  [FiltRef_TJ200FADEC] -> Multiport Switch4/6
  [BoosterRStatus] -> TJ1200 FADEC1/13(Right Booster State)
  [BoosterLStatus] -> TJ1200 FADEC1/12(Left Booster State)
  [SysFaults] -> TJ1200 FADEC1/11(System Faults)
  [OPRPMManual] -> TJ1200 FADEC1/10(Oil Pump RPM Manual Ref)
  TJ1200 FADEC1/8(Closed Loop Model) -> [ClosedLoopModel_TJ200FADEC]
  TJ1200 FADEC1/9(Oil Pump RPM Ref) -> [OPRPM_TJ200FADEC]
  [ExCom] -> TJ1200 FADEC1/9(OnOffCom)
  TJ1200 FADEC1/7(Fuel Lack Model) -> [FuelLackModel_TJ200FADEC]
  TJ1200 FADEC1/6(Normal Model) -> [NormalModel_TJ200FADEC]
  [DigKeys] -> TJ1200 FADEC1/8(Digital Keys)
  [SensFaults] -> TJ1200 FADEC1/7(Sensor Faults)
  [Tt4_HIL] -> Memory11/1
  Memory11/1 -> TJ1200 FADEC1/6(Tt4)  "Tt4"
  Memory10/1 -> TJ1200 FADEC1/5(Sensors)
  [Sensors] -> Memory10/1
  TJ1200 FADEC1/5(FiltRef) -> [FiltRef_TJ200FADEC]
  TJ1200 FADEC1/4(RPMRef) -> [RPMRef_TJ200FADEC]
  [Altitude] -> TJ1200 FADEC1/1(Altitude)
  TJ1200 FADEC1/1(MinMaxWf) -> [Wf_TJ200FADEC], Scope64/1
  [Ref] -> TJ1200 FADEC1/4(RefVecDyn)
  [ControlIn] -> TJ1200 FADEC1/3(Engine Outputs)
  TJ1200 FADEC1/2(Active Controller) -> [Active_TJ200FADEC]
  TJ1200 FADEC1/3(Igniter) -> [Igniter_TJ200FADEC]
  [MN] -> TJ1200 FADEC1/2(MN)
  Interval Test1/1 -> TJ1200 FADEC1/Enable
  [WhichEngine] -> Interval Test1/1
  [OPRPM_TJ200FADEC] -> Multiport Switch16/6
  [OPRPM_TJ700FADEC] -> Multiport Switch16/5
  [ClosedLoopModel_TJ200FADEC] -> Multiport Switch15/6
  [ClosedLoopModel_TJ700FADEC] -> Multiport Switch15/5
  [FuelLackModel_TJ200FADEC] -> Multiport Switch14/6
  [FuelLackModel_TJ700FADEC] -> Multiport Switch14/5
  [NormalModel_TJ200FADEC] -> Multiport Switch13/6
  [NormalModel_TJ700FADEC] -> Multiport Switch13/5
  Multiport Switch16/1 -> [OPRPM_FADEC]
  Multiport Switch13/1 -> [NormalModel_FADEC]
  [ClosedLoopModel_GEJ85FADEC] -> Multiport Switch15/4
  [FuelLackModel_GEJ85FADEC] -> Multiport Switch14/4
  Multiport Switch15/1 -> [ClosedLoopModel_FADEC]
  [FuelLackModel_TF1200FADEC] -> Multiport Switch14/3
  [OPRPM_TF1200FADEC] -> Multiport Switch16/3
  [NormalModel_TJ1200FADEC] -> Multiport Switch13/2
  [NormalModel_GEJ85FADEC] -> Multiport Switch13/4
  [NormalModel_TF1200FADEC] -> Multiport Switch13/3
  [WhichEngine] -> Multiport Switch13/1
  [WhichEngine] -> Multiport Switch15/1
  [WhichEngine] -> Multiport Switch16/1
  [OPRPM_GEJ85FADEC] -> Multiport Switch16/4
  [ClosedLoopModel_TJ1200FADEC] -> Multiport Switch15/2
  [ClosedLoopModel_TF1200FADEC] -> Multiport Switch15/3
  [OPRPM_TJ1200FADEC] -> Multiport Switch16/2
  [FuelLackModel_TJ1200FADEC] -> Multiport Switch14/2
  [WhichEngine] -> Multiport Switch14/1
  Multiport Switch14/1 -> [FuelLackModel_FADEC]
  Constant61/1 -> [NormalModel_TF1200FADEC]
  Constant62/1 -> [NormalModel_GEJ85FADEC]
  Constant63/1 -> [NormalModel_TJ700FADEC]
  Constant66/1 -> [FuelLackModel_GEJ85FADEC]
  Constant65/1 -> [FuelLackModel_TF1200FADEC]
  Constant67/1 -> [FuelLackModel_TJ700FADEC]
  Constant70/1 -> [ClosedLoopModel_GEJ85FADEC]
  Constant69/1 -> [ClosedLoopModel_TF1200FADEC]
  Constant71/1 -> [ClosedLoopModel_TJ700FADEC]
  Constant74/1 -> [OPRPM_GEJ85FADEC]
  Constant73/1 -> [OPRPM_TF1200FADEC]
  Constant75/1 -> [OPRPM_TJ700FADEC]
  Constant52/1 -> [ExtFPModel]
  [ExtFPModel] -> Single Spool Engine/23(External Fuel Pump Model)
  [FlightStart] -> Single Spool Engine/24(Flight Start)
  Constant54/1 -> [FlightStart]
  Constant68/1 -> [FiltRef_TJ40FADEC]
  Constant64/1 -> [RPMRef_TJ40FADEC]
  Constant60/1 -> [Igniter_TJ40FADEC]
  Constant58/1 -> [Active_TJ40FADEC]
  Constant56/1 -> [Wf_TJ40FADEC]
  Constant72/1 -> [NormalModel_TJ40FADEC]
  Constant76/1 -> [FuelLackModel_TJ40FADEC]
  Constant77/1 -> [ClosedLoopModel_TJ40FADEC]
  Constant78/1 -> [OPRPM_TJ40FADEC]
  [Wf_TJ40FADEC] -> Multiport Switch/7
  [Active_TJ40FADEC] -> Multiport Switch1/7
  [Igniter_TJ40FADEC] -> Multiport Switch2/7
  [RPMRef_TJ40FADEC] -> Multiport Switch3/7
  [FiltRef_TJ40FADEC] -> Multiport Switch4/7
  [NormalModel_TJ40FADEC] -> Multiport Switch13/7
  [FuelLackModel_TJ40FADEC] -> Multiport Switch14/7
  [ClosedLoopModel_TJ40FADEC] -> Multiport Switch15/7
  [OPRPM_TJ40FADEC] -> Multiport Switch16/7
  Demux4/4 -> Scope15/2
  [TBearSens0] -> Display/1
  [TBearSens1] -> Display11/1
  [TBearSens2] -> Display12/1

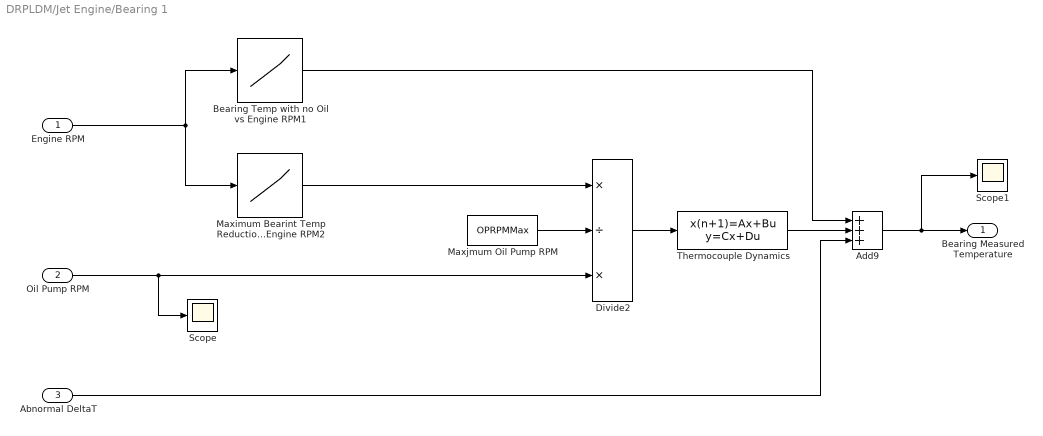
== system DRPLDM/Jet Engine/Bearing 1 ==
  Engine RPM : Inport
  Oil Pump RPM : Inport  Port=2
  Abnormal DeltaT : Inport  Port=3
  Add9 : Sum  Inputs=+++
  Bearing Temp with no Oil vs Engine RPM1 : Lookup_n-D  NumberOfTableDimensions=1  BreakpointsForDimension1=B1ERPM  Table=B1NOOILT  InternalRulePriority=Speed  RndMeth=Simplest  InputSameDT=on
  Divide2 : Product  Inputs=*/*
  Maximum Bearint Temp Reduction at Max Oil Pump RPM vs Engine RPM2 : Lookup_n-D  NumberOfTableDimensions=1  BreakpointsForDimension1=B1ERPM  Table=B1DELTT  InternalRulePriority=Speed  RndMeth=Simplest  InputSameDT=on
  Maxjmum Oil Pump RPM : Constant  Value=OPRPMMax
  Scope : Scope
  Scope1 : Scope
  Thermocouple Dynamics : DiscreteStateSpace  A=Ad  B=Bd  C=Cd  D=Dd  InitialCondition=TBear1Init  SampleTime=Tsim
  Bearing Measured Temperature : Outport
  wires:
  Maximum Bearint Temp Reduction at Max Oil Pump RPM vs Engine RPM2/1 -> Divide2/1
  Divide2/1 -> Thermocouple Dynamics/1
  Thermocouple Dynamics/1 -> Add9/2
  Engine RPM/1 -> Bearing Temp with no Oil vs Engine RPM1/1, Maximum Bearint Temp Reduction at Max Oil Pump RPM vs Engine RPM2/1
  Oil Pump RPM/1 -> Scope/1, Divide2/3
  Bearing Temp with no Oil vs Engine RPM1/1 -> Add9/1
  Maxjmum Oil Pump RPM/1 -> Divide2/2
  Add9/1 -> Scope1/1, Bearing Measured Temperature/1
  Abnormal DeltaT/1 -> Add9/3

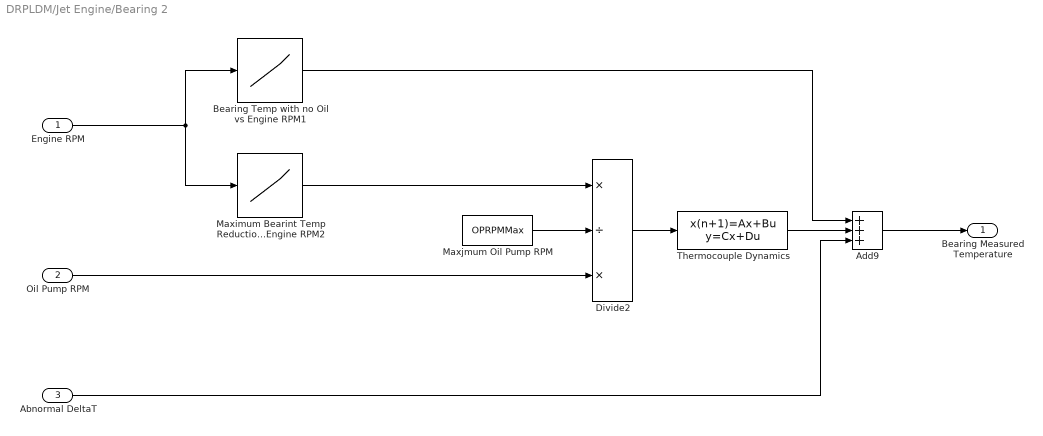
== system DRPLDM/Jet Engine/Bearing 2 ==
  Engine RPM : Inport
  Oil Pump RPM : Inport  Port=2
  Abnormal DeltaT : Inport  Port=3
  Add9 : Sum  Inputs=+++
  Bearing Temp with no Oil vs Engine RPM1 : Lookup_n-D  NumberOfTableDimensions=1  BreakpointsForDimension1=B2ERPM  Table=B2NOOILT  InternalRulePriority=Speed  RndMeth=Simplest  InputSameDT=on
  Divide2 : Product  Inputs=*/*
  Maximum Bearint Temp Reduction at Max Oil Pump RPM vs Engine RPM2 : Lookup_n-D  NumberOfTableDimensions=1  BreakpointsForDimension1=B2ERPM  Table=B2DELTT  InternalRulePriority=Speed  RndMeth=Simplest  InputSameDT=on
  Maxjmum Oil Pump RPM : Constant  Value=OPRPMMax
  Thermocouple Dynamics : DiscreteStateSpace  A=Ad  B=Bd  C=Cd  D=Dd  InitialCondition=TBear2Init  SampleTime=Tsim
  Bearing Measured Temperature : Outport
  wires:
  Abnormal DeltaT/1 -> Add9/3
  Add9/1 -> Bearing Measured Temperature/1
  Maxjmum Oil Pump RPM/1 -> Divide2/2
  Bearing Temp with no Oil vs Engine RPM1/1 -> Add9/1
  Oil Pump RPM/1 -> Divide2/3
  Engine RPM/1 -> Maximum Bearint Temp Reduction at Max Oil Pump RPM vs Engine RPM2/1, Bearing Temp with no Oil vs Engine RPM1/1
  Thermocouple Dynamics/1 -> Add9/2
  Divide2/1 -> Thermocouple Dynamics/1
  Maximum Bearint Temp Reduction at Max Oil Pump RPM vs Engine RPM2/1 -> Divide2/1

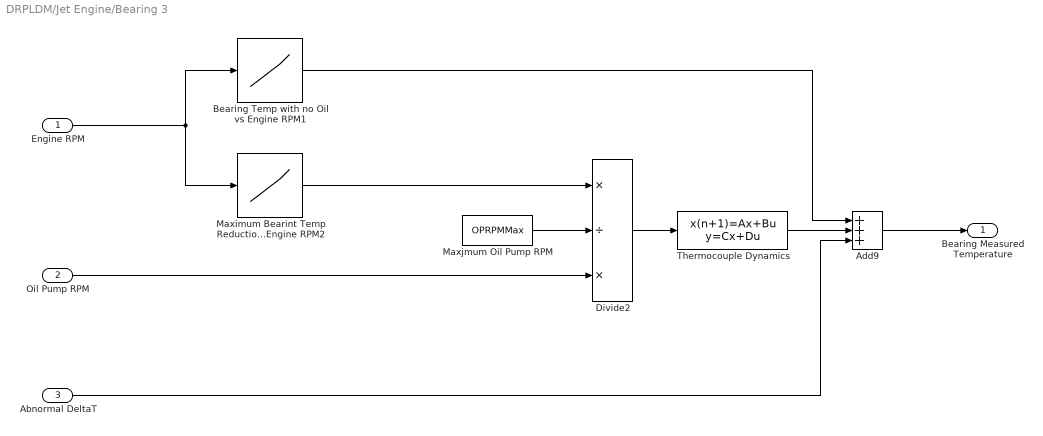
== system DRPLDM/Jet Engine/Bearing 3 ==
  Engine RPM : Inport
  Oil Pump RPM : Inport  Port=2
  Abnormal DeltaT : Inport  Port=3
  Add9 : Sum  Inputs=+++
  Bearing Temp with no Oil vs Engine RPM1 : Lookup_n-D  NumberOfTableDimensions=1  BreakpointsForDimension1=B3ERPM  Table=B3NOOILT  InternalRulePriority=Speed  RndMeth=Simplest  InputSameDT=on
  Divide2 : Product  Inputs=*/*
  Maximum Bearint Temp Reduction at Max Oil Pump RPM vs Engine RPM2 : Lookup_n-D  NumberOfTableDimensions=1  BreakpointsForDimension1=B3ERPM  Table=B3DELTT  InternalRulePriority=Speed  RndMeth=Simplest  InputSameDT=on
  Maxjmum Oil Pump RPM : Constant  Value=OPRPMMax
  Thermocouple Dynamics : DiscreteStateSpace  A=Ad  B=Bd  C=Cd  D=Dd  InitialCondition=TBear3Init  SampleTime=Tsim
  Bearing Measured Temperature : Outport
  wires:
  Maximum Bearint Temp Reduction at Max Oil Pump RPM vs Engine RPM2/1 -> Divide2/1
  Divide2/1 -> Thermocouple Dynamics/1
  Thermocouple Dynamics/1 -> Add9/2
  Engine RPM/1 -> Bearing Temp with no Oil vs Engine RPM1/1, Maximum Bearint Temp Reduction at Max Oil Pump RPM vs Engine RPM2/1
  Oil Pump RPM/1 -> Divide2/3
  Bearing Temp with no Oil vs Engine RPM1/1 -> Add9/1
  Maxjmum Oil Pump RPM/1 -> Divide2/2
  Add9/1 -> Bearing Measured Temperature/1
  Abnormal DeltaT/1 -> Add9/3

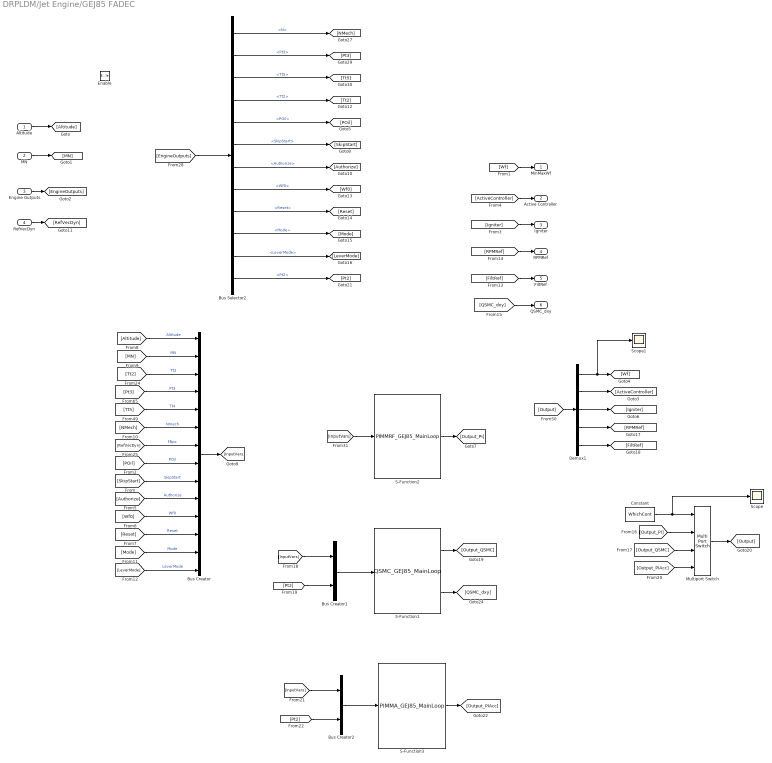
== system DRPLDM/Jet Engine/GEJ85 FADEC ==
  Altitude : Inport
  MN : Inport  Port=2
  Engine Outputs : Inport  Port=3
  RefVecDyn : Inport  Port=4
  Enable : EnablePort
  Bus Creator : BusCreator  Inputs=14
  Bus Creator1 : BusCreator  Inputs=2
  Bus Creator2 : BusCreator  Inputs=2
  Bus Selector2 : BusSelector  OutputSignals=N,Pt3,Tt5,Tt2,POil,SkipStart,Authorize,Wf0,Reset,Mode,LeverMode,Pt2
  Constant : Constant  Value=WhichCont
  Demux1 : Demux  Outputs=5
  Multiport Switch : MultiPortSwitch
  S-Function1 : S-Function  FunctionName=QSMC_GEJ85_MainLoop  SFunctionDeploymentMode=off  EnableBusSupport=off
  S-Function2 : S-Function  FunctionName=PIMMRF_GEJ85_MainLoop  SFunctionDeploymentMode=off  EnableBusSupport=off
  S-Function3 : S-Function  FunctionName=PIMMA_GEJ85_MainLoop  SFunctionDeploymentMode=off  EnableBusSupport=off
  Scope : Scope
  Scope1 : Scope
  MinMaxWf : Outport
  Active Controller : Outport  Port=2  InitialOutput=0
  Igniter : Outport  Port=3  InitialOutput=0
  RPMRef : Outport  Port=4  InitialOutput=0
  FiltRef : Outport  Port=5  InitialOutput=0
  QSMC_dxy : Outport  Port=6  InitialOutput=0
  wires:
  Demux1/5 -> [FiltRef]
  Demux1/4 -> [RPMRef]
  [FiltRef] -> FiltRef/1
  [RPMRef] -> RPMRef/1
  Bus Selector2/4 -> [Tt2]  "<Tt2>"
  Altitude/1 -> [Altitude]
  MN/1 -> [MN]
  Engine Outputs/1 -> [EngineOutputs]
  RefVecDyn/1 -> [RefVecDyn]
  [EngineOutputs] -> Bus Selector2/1
  Bus Selector2/1 -> [NMech]  "<N>"
  Bus Selector2/2 -> [Pt3]  "<Pt3>"
  Bus Selector2/3 -> [Tt5]  "<Tt5>"
  [Wf] -> MinMaxWf/1
  [ActiveController] -> Active Controller/1
  [Altitude] -> Bus Creator/1  "Altitude"
  [MN] -> Bus Creator/2  "MN"
  Bus Creator/1 -> [InputVars]
  [InputVars] -> S-Function2/1
  S-Function2/1 -> [Output_PI]
  [Output] -> Demux1/1
  Demux1/1 -> Scope1/1, [Wf]
  Demux1/2 -> [ActiveController]
  [Tt2] -> Bus Creator/3  "Tt2"
  [Pt3] -> Bus Creator/4  "Pt3"
  [Tt5] -> Bus Creator/5  "Tt4"
  [NMech] -> Bus Creator/6  "Nmech"
  [RefVecDyn] -> Bus Creator/7  "FNpc"
  Bus Selector2/5 -> [POil]  "<POil>"
  [POil] -> Bus Creator/8  "POil"
  Demux1/3 -> [Igniter]
  [Igniter] -> Igniter/1
  Bus Selector2/6 -> [SkipStart]  "<SkipStart>"
  [SkipStart] -> Bus Creator/9  "SkipStart"
  Bus Selector2/7 -> [Authorize]  "<Authorize>"
  Bus Selector2/8 -> [Wf0]  "<Wf0>"
  [Authorize] -> Bus Creator/10  "Authorize"
  [Wf0] -> Bus Creator/11  "Wf0"
  Bus Selector2/9 -> [Reset]  "<Reset>"
  [Reset] -> Bus Creator/12  "Reset"
  Bus Selector2/10 -> [Mode]  "<Mode>"
  Bus Selector2/11 -> [LeverMode]  "<LeverMode>"
  [Mode] -> Bus Creator/13  "Mode"
  [LeverMode] -> Bus Creator/14  "LeverMode"
  Bus Creator1/1 -> S-Function1/1
  S-Function1/1 -> [Output_QSMC]
  [Output_QSMC] -> Multiport Switch/3
  [Output_PI] -> Multiport Switch/2
  Constant/1 -> Scope/1, Multiport Switch/1
  Multiport Switch/1 -> [Output]
  [InputVars] -> Bus Creator1/1
  Bus Selector2/12 -> [Pt2]  "<Pt2>"
  [Pt2] -> Bus Creator1/2
  S-Function1/2 -> [QSMC_dxy]
  [QSMC_dxy] -> QSMC_dxy/1
  S-Function3/1 -> [Output_PIAcc]
  [Pt2] -> Bus Creator2/2
  [InputVars] -> Bus Creator2/1
  Bus Creator2/1 -> S-Function3/1
  [Output_PIAcc] -> Multiport Switch/4

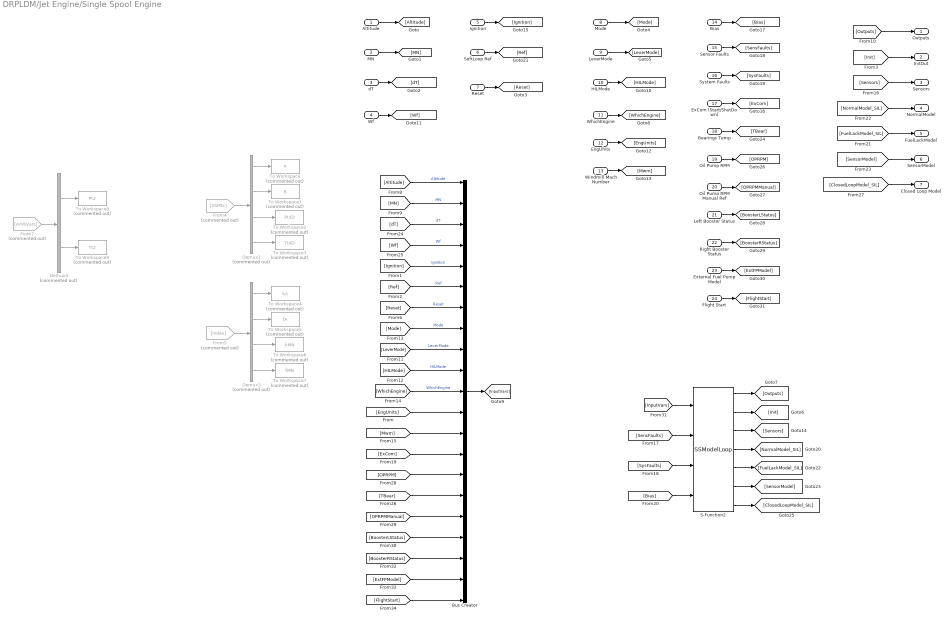
== system DRPLDM/Jet Engine/Single Spool Engine ==
  Altitude : Inport
  MN : Inport  Port=2
  dT : Inport  Port=3
  Wf : Inport  Port=4
  Ignition : Inport  Port=5
  SoftLoop Ref : Inport  Port=6
  Reset : Inport  Port=7
  Mode : Inport  Port=8
  LeverMode : Inport  Port=9
  HILMode : Inport  Port=10
  WhichEngine : Inport  Port=11
  EngUhits : Inport  Port=12
  Windmill Mach Number : Inport  Port=13
  Bias : Inport  Port=14
  Sensor Faults : Inport  Port=15
  System Faults : Inport  Port=16
  ExCom (Start/ShutDown) : Inport  Port=17
  Bearings Temp : Inport  Port=18
  Oil Pump RPM : Inport  Port=19
  Oil Pump RPM Manual Ref : Inport  Port=20
  Left Booster Status : Inport  Port=21
  Right Booster Status : Inport  Port=22
  External Fuel Pump Model : Inport  Port=23
  Flight Start : Inport  Port=24
  Bus Creator : BusCreator  Inputs=21
  Demux1 : Demux  Commented=on
  Demux3 : Demux  Commented=on
  Demux4 : Demux  Commented=on  Outputs=2
  From4 : From  Commented=on  GotoTag=SSMtx
  From5 : From  Commented=on  GotoTag=Index
  From7 : From  Commented=on  GotoTag=AmbVars
  S-Function2 : S-Function  FunctionName=SSModelLoop  SFunctionDeploymentMode=off  EnableBusSupport=off
  To Workspace : ToWorkspace  Commented=on  VariableName=A  SampleTime=-1
  To Workspace1 : ToWorkspace  Commented=on  VariableName=B  SampleTime=-1
  To Workspace2 : ToWorkspace  Commented=on  VariableName=Pt3D  SampleTime=-1
  To Workspace3 : ToWorkspace  Commented=on  VariableName=Tt4D  SampleTime=-1
  To Workspace4 : ToWorkspace  Commented=on  VariableName=kA  SampleTime=-1
  To Workspace5 : ToWorkspace  Commented=on  VariableName=fA  SampleTime=-1
  To Workspace6 : ToWorkspace  Commented=on  VariableName=kMN  SampleTime=-1
  To Workspace7 : ToWorkspace  Commented=on  VariableName=fMN  SampleTime=-1
  To Workspace8 : ToWorkspace  Commented=on  VariableName=Pt2  SampleTime=-1
  To Workspace9 : ToWorkspace  Commented=on  VariableName=Tt2  SampleTime=-1
  Outputs : Outport
  InitOut : Outport  Port=2
  Sensors : Outport  Port=3
  NormalModel : Outport  Port=4
  FuelLackModel : Outport  Port=5
  SensorModel : Outport  Port=6
  Closed Loop Model : Outport  Port=7
  wires:
  Ignition/1 -> [Ignition]
  [Outputs] -> Outputs/1
  Demux4/1 -> To Workspace8/1
  Demux4/2 -> To Workspace9/1
  From7/1 -> Demux4/1
  From5/1 -> Demux3/1
  Demux3/3 -> To Workspace6/1
  Demux3/4 -> To Workspace7/1
  Demux3/2 -> To Workspace5/1
  Demux3/1 -> To Workspace4/1
  From4/1 -> Demux1/1
  Demux1/3 -> To Workspace2/1
  Demux1/4 -> To Workspace3/1
  Demux1/2 -> To Workspace1/1
  Demux1/1 -> To Workspace/1
  Altitude/1 -> [Altitude]
  MN/1 -> [MN]
  dT/1 -> [dT]
  Wf/1 -> [Wf]
  [Altitude] -> Bus Creator/1  "Altitude"
  [MN] -> Bus Creator/2  "MN"
  Bus Creator/1 -> [InputVars]
  [dT] -> Bus Creator/3  "dT"
  [Wf] -> Bus Creator/4  "Wf"
  [Ignition] -> Bus Creator/5  "Ignition"
  [InputVars] -> S-Function2/1
  S-Function2/1 -> [Outputs]
  SoftLoop Ref/1 -> [Ref]
  [Ref] -> Bus Creator/6  "Ref"
  S-Function2/2 -> [Init]
  [Init] -> InitOut/1
  [Reset] -> Bus Creator/7  "Reset"
  Reset/1 -> [Reset]
  WhichEngine/1 -> [WhichEngine]
  HILMode/1 -> [HILMode]
  LeverMode/1 -> [LeverMode]
  Mode/1 -> [Mode]
  [Mode] -> Bus Creator/8  "Mode"
  [LeverMode] -> Bus Creator/9  "LeverMode"
  [HILMode] -> Bus Creator/10  "HILMode"
  [WhichEngine] -> Bus Creator/11  "WhichEngine"
  EngUhits/1 -> [EngUnits]
  [EngUnits] -> Bus Creator/12
  [Mwm] -> Bus Creator/13
  Windmill Mach Number/1 -> [Mwm]
  S-Function2/3 -> [Sensors]
  [Sensors] -> Sensors/1
  [SensFaults] -> S-Function2/2
  [SysFaults] -> S-Function2/3
  Bias/1 -> [Bias]
  System Faults/1 -> [SysFaults]
  Sensor Faults/1 -> [SensFaults]
  [Bias] -> S-Function2/4
  [ExCom] -> Bus Creator/14
  ExCom (Start/ShutDown)/1 -> [ExCom]
  S-Function2/4 -> [NormalModel_SIL]
  S-Function2/5 -> [FuelLackModel_SIL]
  [FuelLackModel_SIL] -> FuelLackModel/1
  [NormalModel_SIL] -> NormalModel/1
  S-Function2/6 -> [SensorModel]
  [SensorModel] -> SensorModel/1
  Bearings Temp/1 -> [TBear]
  [TBear] -> Bus Creator/16
  S-Function2/7 -> [ClosedLoopModel_SIL]
  [ClosedLoopModel_SIL] -> Closed Loop Model/1
  [OPRPM] -> Bus Creator/15
  Oil Pump RPM/1 -> [OPRPM]
  [OPRPMManual] -> Bus Creator/17
  Oil Pump RPM Manual Ref/1 -> [OPRPMManual]
  Right Booster Status/1 -> [BoosterRStatus]
  Left Booster Status/1 -> [BoosterLStatus]
  [BoosterLStatus] -> Bus Creator/18
  [BoosterRStatus] -> Bus Creator/19
  External Fuel Pump Model/1 -> [ExtFPModel]
  [ExtFPModel] -> Bus Creator/20
  [FlightStart] -> Bus Creator/21
  Flight Start/1 -> [FlightStart]

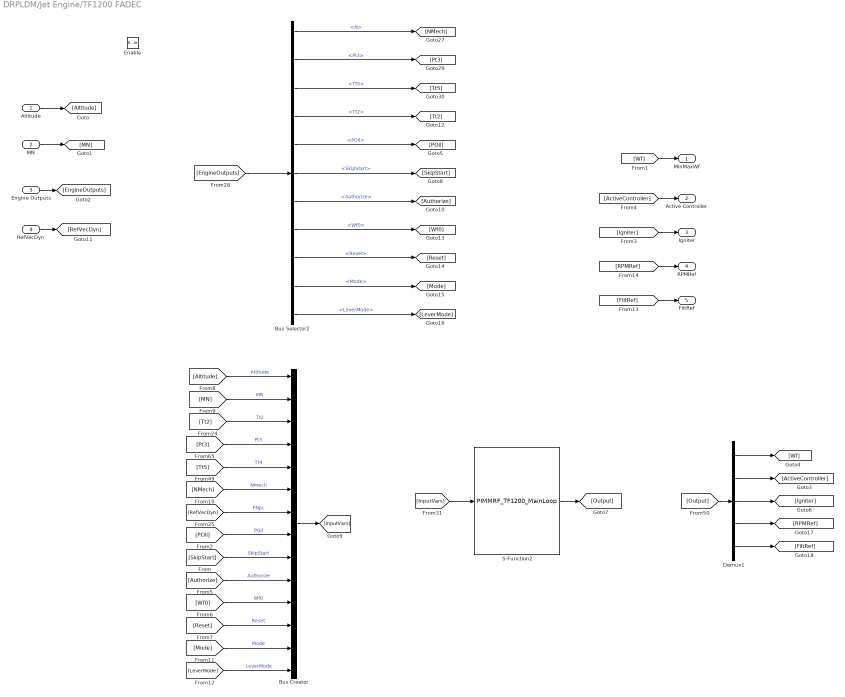
== system DRPLDM/Jet Engine/TF1200 FADEC ==
  Altitude : Inport
  MN : Inport  Port=2
  Engine Outputs : Inport  Port=3
  RefVecDyn : Inport  Port=4
  Enable : EnablePort
  Bus Creator : BusCreator  Inputs=14
  Bus Selector2 : BusSelector  OutputSignals=N,Pt3,Tt5,Tt2,POil,SkipStart,Authorize,Wf0,Reset,Mode,LeverMode
  Demux1 : Demux  Outputs=5
  S-Function2 : S-Function  FunctionName=PIMMRF_TF1200_MainLoop  SFunctionDeploymentMode=off  EnableBusSupport=off
  MinMaxWf : Outport
  Active Controller : Outport  Port=2  InitialOutput=0
  Igniter : Outport  Port=3  InitialOutput=0
  RPMRef : Outport  Port=4  InitialOutput=0
  FiltRef : Outport  Port=5  InitialOutput=0
  wires:
  [LeverMode] -> Bus Creator/14  "LeverMode"
  [Mode] -> Bus Creator/13  "Mode"
  Bus Selector2/11 -> [LeverMode]  "<LeverMode>"
  Bus Selector2/10 -> [Mode]  "<Mode>"
  [Reset] -> Bus Creator/12  "Reset"
  Bus Selector2/9 -> [Reset]  "<Reset>"
  [Wf0] -> Bus Creator/11  "Wf0"
  [Authorize] -> Bus Creator/10  "Authorize"
  Bus Selector2/8 -> [Wf0]  "<Wf0>"
  Bus Selector2/7 -> [Authorize]  "<Authorize>"
  [SkipStart] -> Bus Creator/9  "SkipStart"
  Bus Selector2/6 -> [SkipStart]  "<SkipStart>"
  [Igniter] -> Igniter/1
  Demux1/3 -> [Igniter]
  [POil] -> Bus Creator/8  "POil"
  Bus Selector2/5 -> [POil]  "<POil>"
  [RefVecDyn] -> Bus Creator/7  "FNpc"
  [NMech] -> Bus Creator/6  "Nmech"
  [Tt5] -> Bus Creator/5  "Tt4"
  [Pt3] -> Bus Creator/4  "Pt3"
  [Tt2] -> Bus Creator/3  "Tt2"
  Demux1/2 -> [ActiveController]
  Demux1/1 -> [Wf]
  [Output] -> Demux1/1
  S-Function2/1 -> [Output]
  [InputVars] -> S-Function2/1
  Bus Creator/1 -> [InputVars]
  [MN] -> Bus Creator/2  "MN"
  [Altitude] -> Bus Creator/1  "Altitude"
  [ActiveController] -> Active Controller/1
  [Wf] -> MinMaxWf/1
  Bus Selector2/3 -> [Tt5]  "<Tt5>"
  Bus Selector2/2 -> [Pt3]  "<Pt3>"
  Bus Selector2/1 -> [NMech]  "<N>"
  [EngineOutputs] -> Bus Selector2/1
  RefVecDyn/1 -> [RefVecDyn]
  Engine Outputs/1 -> [EngineOutputs]
  MN/1 -> [MN]
  Altitude/1 -> [Altitude]
  Bus Selector2/4 -> [Tt2]  "<Tt2>"
  [RPMRef] -> RPMRef/1
  [FiltRef] -> FiltRef/1
  Demux1/4 -> [RPMRef]
  Demux1/5 -> [FiltRef]
